simulink model "basic_simulink"  (R2013b)
settings: Solver=ode45  StartTime=0.0  StopTime=10.0  MaxStep=0.1  RelTol=1e-3
settings Model: Creator=aksha  LastModifiedBy=aksha

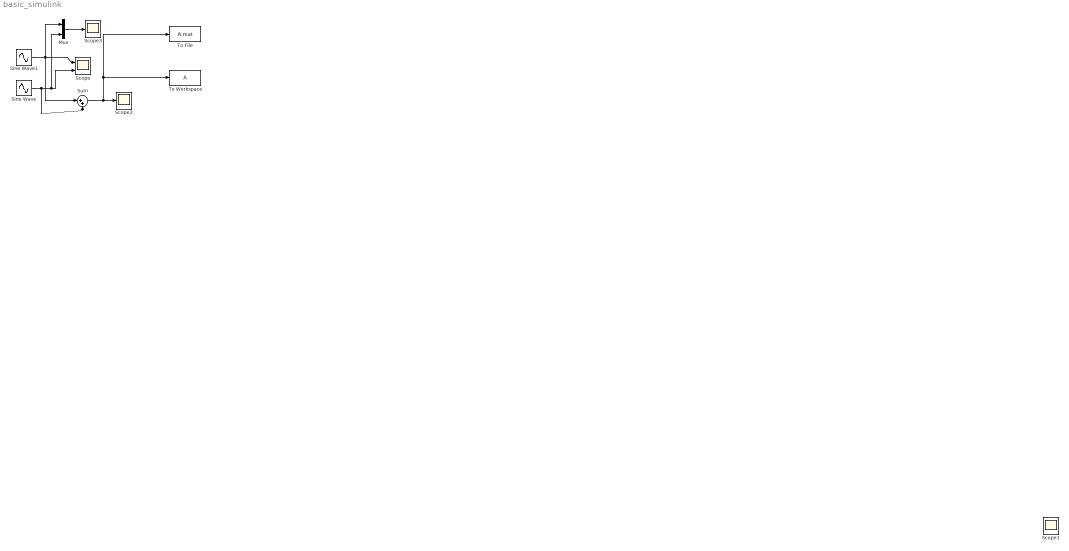
== system basic_simulink ==
  Mux : Mux  Inputs=2
  Scope : Scope  NumInputPorts=2
      settings: YMin=-5~-5  YMax=5~5
  Scope1 : Scope
  Scope2 : Scope
      settings: SaveName=ScopeData2
  Scope3 : Scope
      settings: SaveName=ScopeData3
  Sine Wave : Sin  Amplitude=5  Frequency=2  SampleTime=0
  Sine Wave1 : Sin  Amplitude=2  SampleTime=0
  Sum : Sum  Inputs=|++
  To File : ToFile  Filename=A.mat  MatrixName=A  SaveFormat=Timeseries
  To Workspace : ToWorkspace  VariableName=A  SampleTime=-1  SaveFormat=Timeseries
  wires:
  Sine Wave1/1 -> Mux/1, Sum/1, Scope/1
  Sine Wave/1 -> Sum/2, Mux/2, Scope/2
  Sum/1 -> To File/1, To Workspace/1, Scope2/1
  Mux/1 -> Scope3/1
